simulink model "controller"  (R2022a)
settings: Solver=VariableStepAuto  StartTime=0.0  StopTime=1  RelTol=1e-3
libraries: fod x2
settings Model: Creator=user  LastModifiedBy=Jagadeesh

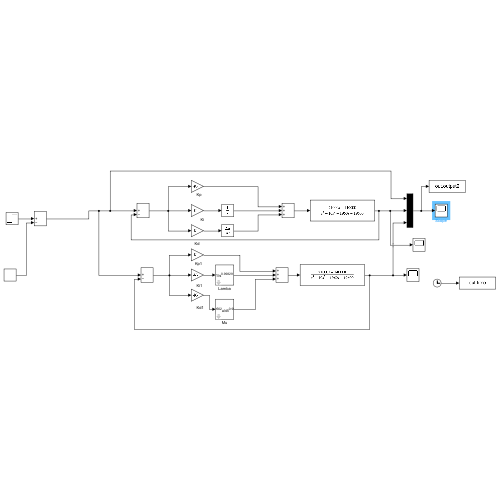
[thumbnail: Simulink's stored preview of the top-level diagram]
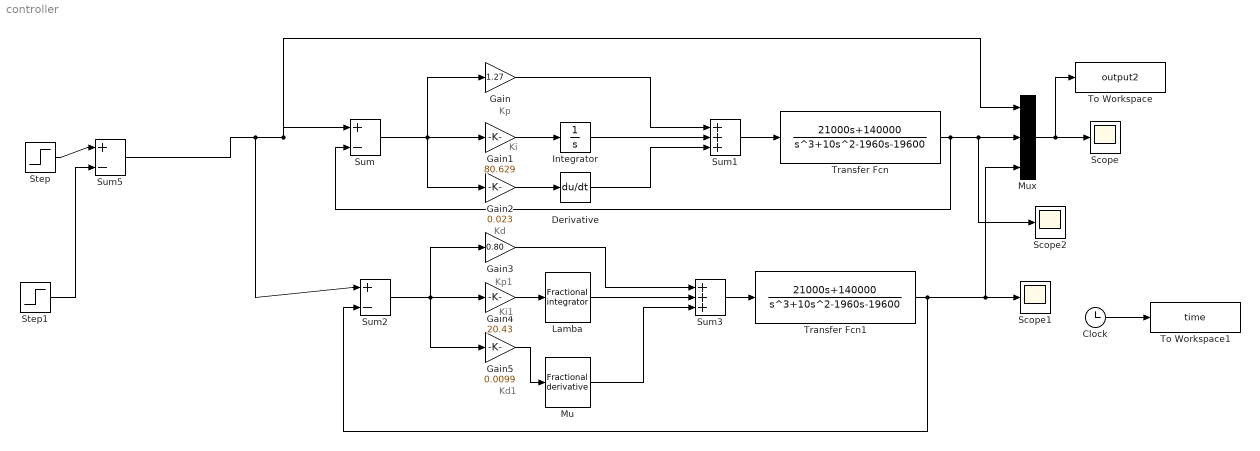
== system controller ==
  note: Kp
  note: Ki
  note: Kd
  note: Kp1
  note: Ki1
  note: Kd1
  Clock : Clock
  Derivative : Derivative
  Gain : Gain  Gain=1.27
  Gain1 : Gain  Gain=80.629
  Gain2 : Gain  Gain=0.023
  Gain3 : Gain  Gain=0.80
  Gain4 : Gain  Gain=20.43
  Gain5 : Gain  Gain=0.0099
  Integrator : Integrator
  Lamba : fod/Fractional integrator  gam=0.998293  ww=[0.001; 1000]  n=5  nFod=off
      settings: SourceProductName=FOMCON Toolbox
  Mu : fod/Fractional derivative  gam=0.99562  ww=[0.001; 1000]  n=1  nFod=off
      settings: SourceProductName=FOMCON Toolbox
  Mux : Mux  Inputs=3
  Scope : Scope
  Scope1 : Scope
  Scope2 : Scope
  Step : Step  Time=0  After=0.5  SampleTime=0
  Step1 : Step  Time=0.5  After=0.3  SampleTime=0
  Sum : Sum  Inputs=|+-
  Sum1 : Sum  Inputs=+++
  Sum2 : Sum  Inputs=|+-
  Sum3 : Sum  Inputs=+++
  Sum5 : Sum  Inputs=|+-
  To Workspace : ToWorkspace  VariableName=output2  SampleTime=-1
  To Workspace1 : ToWorkspace  VariableName=time  SampleTime=-1
  Transfer Fcn : TransferFcn  Numerator=[21000 140000]  Denominator=[1 10 -1960 -19600]
  Transfer Fcn1 : TransferFcn  Numerator=[21000 140000]  Denominator=[1 10 -1960 -19600]
  wires:
  Sum/1 -> Gain/1, Gain2/1, Gain1/1
  Gain1/1 -> Integrator/1
  Gain2/1 -> Derivative/1
  Gain/1 -> Sum1/1
  Integrator/1 -> Sum1/2
  Derivative/1 -> Sum1/3
  Sum1/1 -> Transfer Fcn/1
  Sum2/1 -> Gain3/1, Gain5/1, Gain4/1
  Sum3/1 -> Transfer Fcn1/1
  Gain3/1 -> Sum3/1
  Gain4/1 -> Lamba/1
  Lamba/1 -> Sum3/2
  Gain5/1 -> Mu/1
  Mu/1 -> Sum3/3
  Transfer Fcn/1 -> Sum/2, Scope2/1, Mux/2
  Transfer Fcn1/1 -> Sum2/2, Scope1/1, Mux/3
  Mux/1 -> To Workspace/1, Scope/1
  Clock/1 -> To Workspace1/1
  Step/1 -> Sum5/1
  Step1/1 -> Sum5/2
  Sum5/1 -> Sum2/1, Mux/1, Sum/1
